simulink model "example_multilateration"  (R2016a)
settings: Solver=VariableStepAuto  StartTime=0.0  StopTime=25  RelTol=1e-3
undefined symbols (not defined in the file): inner_h, k, TDOAparam
libraries: dspsrcs4 x6, vrlib x2
settings Model: Creator=Daniel  LastModifiedBy=mgreiff
settings DataIOCC: LimitDataPoints=on
settings DebuggingCC: AllowSymbolicDim=off
settings ModelReferenceCC: PropagateSignalLabelsOutOfModel=off
settings GRTTargetCC: GeneratePreprocessorConditionals=Use local settings

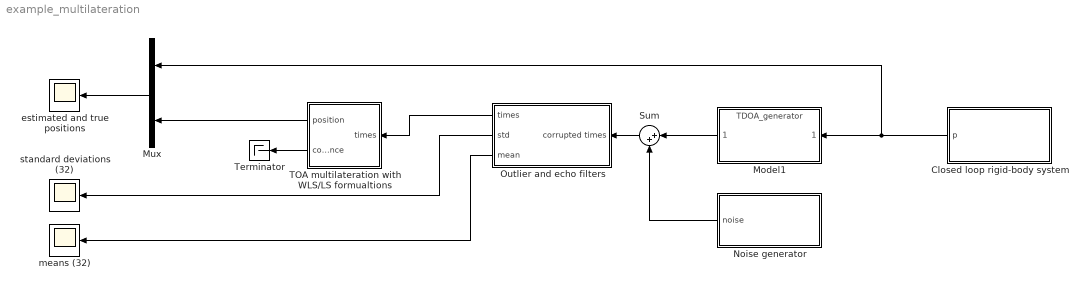
== system example_multilateration ==
  Closed loop rigid-body system : Subsystem
  Model1 : ModelReference  ModelNameDialog=TDOA_generator.slx  SimulationMode=Normal  ModelReferenceVersion=1.3
  Mux : Mux  Inputs=2
  Noise generator : Subsystem
  Outlier and echo filters : Subsystem
  Sum : Sum  Inputs=|++
  TOA multilateration with WLS/LS formualtions : Subsystem
  Terminator : Terminator
  estimated and true positions : Scope
  means (32) : Scope
  standard deviations (32) : Scope
  wires:
  Sum/1 -> Outlier and echo filters/1(corrupted times)
  Outlier and echo filters/2(std) -> standard deviations (32)/1
  Outlier and echo filters/3(mean) -> means (32)/1
  Outlier and echo filters/1(times) -> TOA multilateration with WLS/LS formualtions/1(times)
  TOA multilateration with WLS/LS formualtions/2(confidence) -> Terminator/1
  Closed loop rigid-body system/1(p) -> Mux/1, Model1/1
  Mux/1 -> estimated and true positions/1
  TOA multilateration with WLS/LS formualtions/1(position) -> Mux/2
  Noise generator/1(noise) -> Sum/2
  Model1/1 -> Sum/1

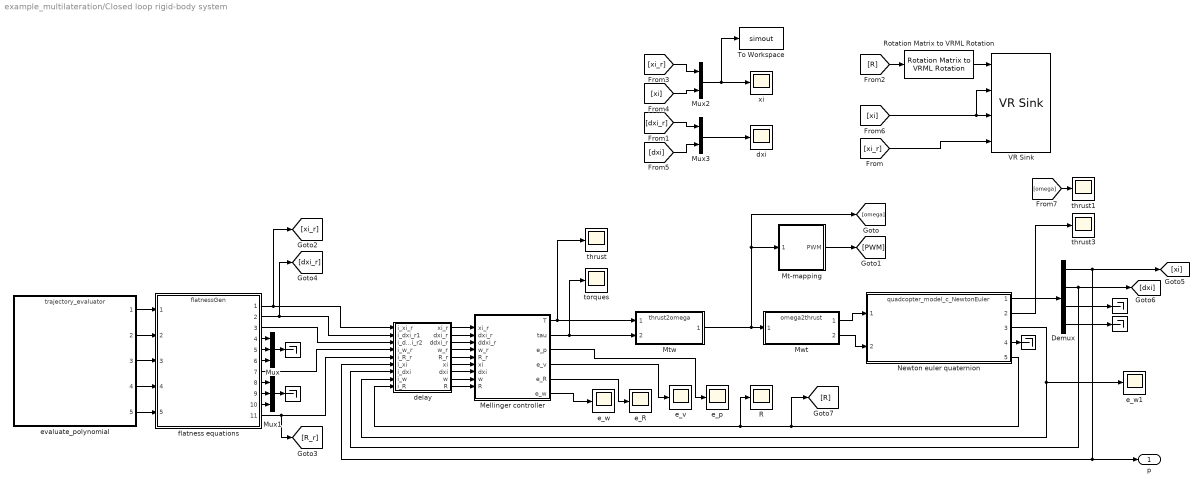
== system example_multilateration/Closed loop rigid-body system ==
  " " : Terminator
  "  " : Terminator
  "     " : Terminator
  "      " : Terminator
  "       " : Terminator
  Demux : Demux  Outputs=[3,3,3,3]
  Mellinger controller : MATLAB Function  TreatAsAtomicUnit=on  SystemSampleTime=inner_h
  Mt-mapping : Subsystem
  Mtw : ModelReference  ModelNameDialog=thrust2omega.mdl  SimulationMode=Normal  ModelReferenceVersion=1.3
  Mux : Mux  Inputs=3
  Mux1 : Mux  Inputs=3
  Mux2 : Mux  Inputs=2
  Mux3 : Mux  Inputs=2
  Mwt : ModelReference  ModelNameDialog=omega2thrust.mdl  SimulationMode=Normal  ModelReferenceVersion=1.3
  Newton euler quaternion : ModelReference  ModelNameDialog=quadcopter_model_c_NewtonEuler.mdl  SimulationMode=Normal  ModelReferenceVersion=1.325
  R : Scope
  Rotation Matrix to VRML Rotation : vrlib/Utilities/Rotation Matrix to VRML Rotation  maxzero=1e-12
  To Workspace : ToWorkspace  VariableName=simout  SaveFormat=Timeseries  SampleTime=-1
  VR Sink : vrlib/VR Sink  InstantiateOnLoad=on  SampleTime=0.05  ViewEnable=on  RemoteChange=off  RemoteView=off  FieldsWritten=copter.rotation.4.1.1.double#copter.translation.3.1.1.double#vp.translation.3.1.1.double#target.translation.3.1.1.double  WorldFileName=copter_world.wrl  WorldDescription=quadcopter_world  AutoView=on  VideoDimensions=[]  AllowVariableSize=off
  delay : Subsystem
  dxi : Scope
  e_R : Scope
  e_p : Scope
  e_v : Scope
  e_w : Scope
  e_w1 : Scope
  evaluate_polynomial : ModelReference  ModelNameDialog=trajectory_evaluator.slx  SimulationMode=Normal  ModelReferenceVersion=1.106
  flatness equations : ModelReference  ModelNameDialog=flatnessGen.slx  SimulationMode=Normal  ModelReferenceVersion=1.117
  thrust : Scope
  thrust1 : Scope
  thrust3 : Scope
  torques : Scope
  xi : Scope
  p : Outport
  wires:
  Demux/4 -> "       "/1
  flatness equations/2 -> delay/2(i_dxi_r1), [dxi_r]
  [xi] -> Mux2/2
  Mux3/1 -> dxi/1
  flatness equations/10 -> Mux1/3
  Mwt/1 -> Newton euler quaternion/1
  Mt-mapping/1(PWM) -> [PWM]
  Mellinger controller/2(tau) -> torques/1, Mtw/2
  delay/7(dxi) -> Mellinger controller/7(dxi)
  evaluate_polynomial/5 -> flatness equations/5
  delay/4(w_r) -> Mellinger controller/4(w_r)
  delay/9(R) -> Mellinger controller/9(R)
  flatness equations/4 -> Mux/1
  delay/3(ddxi_r) -> Mellinger controller/3(ddxi_r)
  delay/1(xi_r) -> Mellinger controller/1(xi_r)
  flatness equations/7 -> delay/4(i_w_r)
  [R] -> Rotation Matrix to VRML Rotation/1
  Mwt/2 -> Newton euler quaternion/2
  evaluate_polynomial/4 -> flatness equations/4
  [dxi] -> Mux3/2
  Mux2/1 -> To Workspace/1, xi/1
  Mux1/1 -> "  "/1
  [xi_r] -> VR Sink/4
  Demux/3 -> "      "/1
  delay/5(R_r) -> Mellinger controller/5(R_r)
  delay/6(xi) -> Mellinger controller/6(xi)
  Newton euler quaternion/5 -> [R], delay/9(i_R), R/1
  Newton euler quaternion/4 -> "     "/1
  evaluate_polynomial/2 -> flatness equations/2
  [dxi_r] -> Mux3/1
  evaluate_polynomial/1 -> flatness equations/1
  Demux/1 -> delay/6(i_xi), p/1, [xi]
  evaluate_polynomial/3 -> flatness equations/3
  Mtw/1 -> Mt-mapping/1(omega), [omega], Mwt/1
  flatness equations/11 -> delay/5(i_R_r), [R_r]
  flatness equations/9 -> Mux1/2
  Newton euler quaternion/1 -> Demux/1
  delay/2(dxi_r) -> Mellinger controller/2(dxi_r)
  Rotation Matrix to VRML Rotation/1 -> VR Sink/1
  Mellinger controller/3(e_p) -> e_p/1
  flatness equations/1 -> delay/1(i_xi_r), [xi_r]
  Newton euler quaternion/3 -> e_w1/1, delay/8(i_w)
  flatness equations/5 -> Mux/2
  delay/8(w) -> Mellinger controller/8(w)
  Mellinger controller/1(T) -> Mtw/1, thrust/1
  Mellinger controller/4(e_v) -> e_v/1
  flatness equations/3 -> delay/3(i_ddxi_r2)
  Newton euler quaternion/2 -> thrust3/1
  Mellinger controller/6(e_w) -> e_w/1
  Demux/2 -> delay/7(i_dxi), [dxi]
  Mellinger controller/5(e_R) -> e_R/1
  flatness equations/6 -> Mux/3
  [xi_r] -> Mux2/1
  [xi] -> VR Sink/2, VR Sink/3
  Mux/1 -> " "/1
  [omega] -> thrust1/1
  flatness equations/8 -> Mux1/1

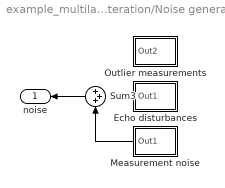
== system example_multilateration/Noise generator ==
  Echo disturbances : Subsystem
  Measurement noise : Subsystem
  Outlier measurements : Subsystem
  Sum3 : Sum  Inputs=+++
  noise : Outport
  wires:
  Sum3/1 -> noise/1
  Measurement noise/1(Out1) -> Sum3/3

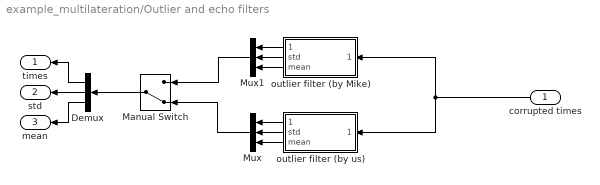
== system example_multilateration/Outlier and echo filters ==
  corrupted times : Inport
  Demux : Demux  Outputs=[6,6,6]
  Manual Switch : ManualSwitch  CurrentSetting=0
  Mux : Mux  Inputs=3
  Mux1 : Mux  Inputs=3
  outlier filter (by Mike) : Subsystem  TreatAsAtomicUnit=on  SystemSampleTime=1/60
  outlier filter (by us) : Subsystem  TreatAsAtomicUnit=on  SystemSampleTime=1/60
  times : Outport
  std : Outport  Port=2
  mean : Outport  Port=3
  wires:
  corrupted times/1 -> outlier filter (by us)/1(tm_tdoa), outlier filter (by Mike)/1(tm_tdoa)
  Manual Switch/1 -> Demux/1
  Mux1/1 -> Manual Switch/1
  outlier filter (by Mike)/1(tf_tdoa) -> Mux1/1
  outlier filter (by Mike)/2(std) -> Mux1/2
  outlier filter (by Mike)/3(mean) -> Mux1/3
  outlier filter (by us)/1(tf_tdoa) -> Mux/1
  outlier filter (by us)/2(std) -> Mux/2
  outlier filter (by us)/3(mean) -> Mux/3
  Mux/1 -> Manual Switch/2
  Demux/3 -> mean/1
  Demux/2 -> std/1
  Demux/1 -> times/1

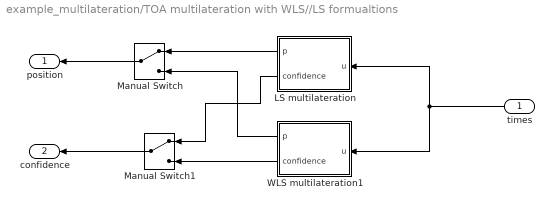
== system example_multilateration/TOA multilateration with WLS//LS formualtions ==
  times : Inport  PortDimensions=6
  LS multilateration : MATLAB Function  TreatAsAtomicUnit=on
  Manual Switch : ManualSwitch
  Manual Switch1 : ManualSwitch
  WLS multilateration1 : MATLAB Function  TreatAsAtomicUnit=on
  position : Outport  PortDimensions=3
  confidence : Outport  Port=2  PortDimensions=3
  wires:
  Manual Switch/1 -> position/1
  times/1 -> WLS multilateration1/1(u), LS multilateration/1(u)
  LS multilateration/1(p) -> Manual Switch/1
  WLS multilateration1/1(p) -> Manual Switch/2
  LS multilateration/2(confidence) -> Manual Switch1/1
  Manual Switch1/1 -> confidence/1
  WLS multilateration1/2(confidence) -> Manual Switch1/2

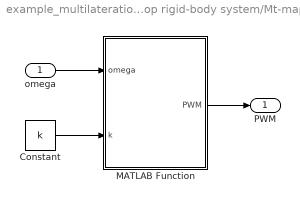
== system example_multilateration/Closed loop rigid-body system/Mt-mapping ==
  omega : Inport
  Constant : Constant  Value=k
  MATLAB Function : MATLAB Function  TreatAsAtomicUnit=on
  PWM : Outport
  wires:
  MATLAB Function/1(PWM) -> PWM/1
  omega/1 -> MATLAB Function/1(omega)
  Constant/1 -> MATLAB Function/2(k)

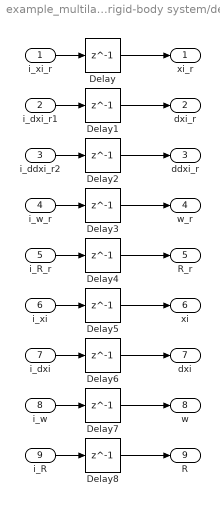
== system example_multilateration/Closed loop rigid-body system/delay ==
  i_xi_r : Inport
  i_dxi_r1 : Inport  Port=2
  i_ddxi_r2 : Inport  Port=3
  i_w_r : Inport  Port=4
  i_R_r : Inport  Port=5
  i_xi : Inport  Port=6
  i_dxi : Inport  Port=7
  i_w : Inport  Port=8
  i_R : Inport  Port=9
  Delay{,1..8} (9 alike) : Delay  DelayLength=1  InitialCondition=0  SampleTime=inner_h
  xi_r : Outport
  dxi_r : Outport  Port=2
  ddxi_r : Outport  Port=3
  w_r : Outport  Port=4
  R_r : Outport  Port=5
  xi : Outport  Port=6
  dxi : Outport  Port=7
  w : Outport  Port=8
  R : Outport  Port=9
  wires:
  Delay/1 -> xi_r/1
  Delay1/1 -> dxi_r/1
  Delay2/1 -> ddxi_r/1
  Delay4/1 -> R_r/1
  Delay3/1 -> w_r/1
  Delay5/1 -> xi/1
  Delay6/1 -> dxi/1
  Delay8/1 -> R/1
  Delay7/1 -> w/1
  i_xi_r/1 -> Delay/1
  i_ddxi_r2/1 -> Delay2/1
  i_dxi_r1/1 -> Delay1/1
  i_w_r/1 -> Delay3/1
  i_R_r/1 -> Delay4/1
  i_xi/1 -> Delay5/1
  i_dxi/1 -> Delay6/1
  i_w/1 -> Delay7/1
  i_R/1 -> Delay8/1

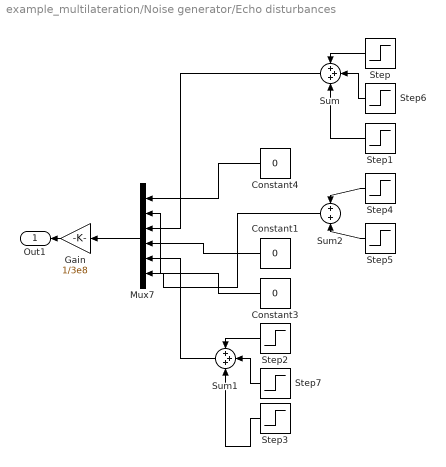
== system example_multilateration/Noise generator/Echo disturbances ==
  Constant1 : Constant  Value=0
  Constant3 : Constant  Value=0
  Constant4 : Constant  Value=0
  Gain : Gain  Gain=1/3e8
  Mux7 : Mux  Inputs=6
  Step : Step  Time=10  After=-0.3  SampleTime=0
  Step1 : Step  Time=14  After=-0.4  SampleTime=0
  Step2 : Step  Time=16  After=0.4  SampleTime=0
  Step3 : Step  Time=22  After=-1  SampleTime=0
  Step4 : Step  Time=3  After=0.3  SampleTime=0
  Step5 : Step  Time=6  After=-0.3  SampleTime=0
  Step6 : Step  Time=12  After=0.7  SampleTime=0
  Step7 : Step  Time=20  After=0.6  SampleTime=0
  Sum : Sum  Inputs=+++
  Sum1 : Sum  Inputs=+++
  Sum2 : Sum  Inputs=+|+
  Out1 : Outport
  wires:
  Step2/1 -> Sum1/1
  Step3/1 -> Sum1/3
  Gain/1 -> Out1/1
  Mux7/1 -> Gain/1
  Step/1 -> Sum/1
  Sum/1 -> Mux7/3
  Constant4/1 -> Mux7/1
  Sum1/1 -> Mux7/5
  Constant3/1 -> Mux7/4
  Constant1/1 -> Mux7/2
  Sum2/1 -> Mux7/6
  Step4/1 -> Sum2/1
  Step5/1 -> Sum2/2
  Step1/1 -> Sum/3
  Step6/1 -> Sum/2
  Step7/1 -> Sum1/2

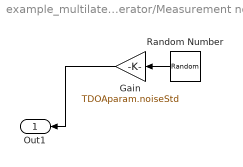
== system example_multilateration/Noise generator/Measurement noise ==
  Gain : Gain  Gain=TDOAparam.noiseStd
  Random Number : RandomNumber  Mean=TDOAparam.noiseMean  Variance=[1,1,1,1,1,1]  SampleTime=1/60
  Out1 : Outport
  wires:
  Gain/1 -> Out1/1
  Random Number/1 -> Gain/1

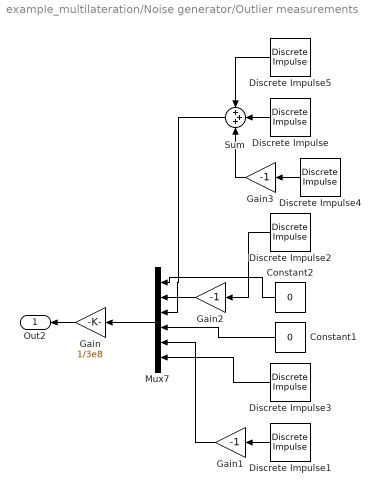
== system example_multilateration/Noise generator/Outlier measurements ==
  Constant1 : Constant  Value=0
  Constant2 : Constant  Value=0
  Discrete Impulse : dspsrcs4/Discrete  Impulse  Delay=700  SampleTime=1/60  FrameSample=1  OutputFrames=off  dataType=double  isSigned=on  wordLen=16  udDataType=sfix(16)  fracBitsMode=Best precision  numFracBits=15  OutDataTypeStr=double  LastOutDataTypeStr=double
  Discrete Impulse1 : dspsrcs4/Discrete  Impulse  Delay=400  SampleTime=1/60  FrameSample=1  OutputFrames=off  dataType=double  isSigned=on  wordLen=16  udDataType=sfix(16)  fracBitsMode=Best precision  numFracBits=15  OutDataTypeStr=double  LastOutDataTypeStr=double
  Discrete Impulse2 : dspsrcs4/Discrete  Impulse  Delay=1000  SampleTime=1/60  FrameSample=1  OutputFrames=off  dataType=double  isSigned=on  wordLen=16  udDataType=sfix(16)  fracBitsMode=Best precision  numFracBits=15  OutDataTypeStr=double  LastOutDataTypeStr=double
  Discrete Impulse3 : dspsrcs4/Discrete  Impulse  Delay=5000  SampleTime=1/60  FrameSample=1  OutputFrames=off  dataType=double  isSigned=on  wordLen=16  udDataType=sfix(16)  fracBitsMode=Best precision  numFracBits=15  OutDataTypeStr=double  LastOutDataTypeStr=double
  Discrete Impulse4 : dspsrcs4/Discrete  Impulse  Delay=800  SampleTime=1/60  FrameSample=1  OutputFrames=off  dataType=double  isSigned=on  wordLen=16  udDataType=sfix(16)  fracBitsMode=Best precision  numFracBits=15  OutDataTypeStr=double  LastOutDataTypeStr=double
  Discrete Impulse5 : dspsrcs4/Discrete  Impulse  Delay=300  SampleTime=1/60  FrameSample=1  OutputFrames=off  dataType=double  isSigned=on  wordLen=16  udDataType=sfix(16)  fracBitsMode=Best precision  numFracBits=15  OutDataTypeStr=double  LastOutDataTypeStr=double
  Gain : Gain  Gain=1/3e8
  Gain1 : Gain  Gain=-1
  Gain2 : Gain  Gain=-1
  Gain3 : Gain  Gain=-1
  Mux7 : Mux  Inputs=6
  Sum : Sum  Inputs=+++
  Out2 : Outport
  wires:
  Gain/1 -> Out2/1
  Discrete Impulse1/1 -> Gain1/1
  Discrete Impulse3/1 -> Mux7/6
  Constant2/1 -> Mux7/1
  Mux7/1 -> Gain/1
  Constant1/1 -> Mux7/4
  Gain1/1 -> Mux7/5
  Gain2/1 -> Mux7/2
  Discrete Impulse2/1 -> Gain2/1
  Discrete Impulse/1 -> Sum/2
  Discrete Impulse4/1 -> Gain3/1
  Discrete Impulse5/1 -> Sum/1
  Sum/1 -> Mux7/3
  Gain3/1 -> Sum/3

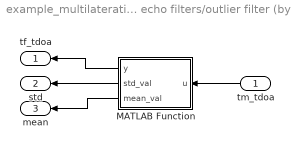
== system example_multilateration/Outlier and echo filters/outlier filter (by Mike) ==
  tm_tdoa : Inport  PortDimensions=6
  MATLAB Function : MATLAB Function  TreatAsAtomicUnit=on
  tf_tdoa : Outport  PortDimensions=6
  std : Outport  Port=2  PortDimensions=6
  mean : Outport  Port=3  PortDimensions=6
  wires:
  MATLAB Function/1(y) -> tf_tdoa/1
  tm_tdoa/1 -> MATLAB Function/1(u)
  MATLAB Function/3(mean_val) -> mean/1
  MATLAB Function/2(std_val) -> std/1

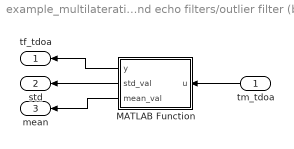
== system example_multilateration/Outlier and echo filters/outlier filter (by us) ==
  tm_tdoa : Inport  PortDimensions=6
  MATLAB Function : MATLAB Function  TreatAsAtomicUnit=on
  tf_tdoa : Outport  PortDimensions=6
  std : Outport  Port=2  PortDimensions=6
  mean : Outport  Port=3  PortDimensions=6
  wires:
  MATLAB Function/1(y) -> tf_tdoa/1
  tm_tdoa/1 -> MATLAB Function/1(u)
  MATLAB Function/3(mean_val) -> mean/1
  MATLAB Function/2(std_val) -> std/1

== matlab function example_multilateration/Outlier and echo filters/outlier filter (by Mike)/MATLAB Function ==
  data: u input; y output; std_val output; mean_val output
function [y, std_val, mean_val] = fcn(u)
persistent TDOA_last_feasible_measurement;
persistent TDOA_series;
if isempty(TDOA_series);
    TDOA_series = zeros(32, 6);
    TDOA_last_feasible_measurement = u;
    disp('here')
end

% Shift TDOA_series such that the most recent measurement is at a low row
% index
TDOA_series(2:end,:) = TDOA_series(1:end-1,:);
TDOA_series(1,:) = u';

series = [];
% Check if the TDOA series contains NaN (cant due ti variable length issues
% in mean() and std())
% if sum(sum(isnan(TDOA_series))) > 0
%     [row, ~] = find(isnan(TDOA_series)); % First column index with NaN
%     series = TDOA_series(1:row(1) - 1, :);
% else
%     series = TDOA_series;
% end

% Compute standard deviation and mean of series;
%if size(series, 1) == 1
std_val = std(TDOA_series);
mean_val = mean(TDOA_series);
   
%end

% 
std_lim = 4;
for ii = 1:length(std_val)
    if std_val(ii)*std_lim >= abs(u(ii) - mean_val(ii))
        TDOA_last_feasible_measurement(ii) = u(ii);
    end
end
y = TDOA_last_feasible_measurement;

== matlab function example_multilateration/Closed loop rigid-body system/Mellinger controller ==
  data: xi_r input; dxi_r input; ddxi_r input; w_r input; R_r input; xi input; T output; tau output; dxi input; w input; R input; e_p output; e_v output; e_R output; e_w output
function [T, tau, e_p, e_v, e_R, e_w] = controller(xi_r, dxi_r, ddxi_r, w_r, R_r, xi, dxi, w, R)
%I = [0.0820; 0.0845; 0.1377];
%A=[0;0;0]
%m = 4.34;

m = 0.027;
g = 9.81;
% Functional tuning for type A
K_p = 0.2 * eye(3);
K_v = 0.025 * eye(3);
K_R = 0.1 * eye(3);
K_w = 0.001 * eye(3);

% Functional tuning for type B
K_p = 0.4 * eye(3);
K_v = 0.1* eye(3);
K_R = 0.4 * eye(3);
K_w = 0.01 * eye(3);

K_p = 0.8 * eye(3);
K_v = 0.12* eye(3);
K_R = 0.5 * eye(3);
K_w = 0.005 * eye(3);

%#codegen
zw = [0; 0; 1];
zb = R(:,3);

e_p = xi_r - xi;
e_v = dxi_r - dxi;
F_des = K_p * e_p + K_v * e_v + m * g * zw + m * ddxi_r;
T = F_des'*zb;

zb_des = F_des./ norm(F_des);
psi = 0;
yc_des = [cos(psi+pi/2); sin(psi+pi/2); 0];
xb_des = cross(yc_des, zb_des)./norm(cross(yc_des, zb_des));
yb_des = cross(zb_des, xb_des);
R_des = [xb_des, yb_des, zb_des];

Ssym = 0.5.* (R_des' * R - R' * R_des);
e_R = -[Ssym(3,2); Ssym(1,3); Ssym(2,1)]; % Vee map
e_w = (w_r - w);

%disp([norm(e_p), norm(e_v), norm(e_R), norm(e_w)])

tau = K_R * e_R + K_w * e_w;

== matlab function example_multilateration/Closed loop rigid-body system/Mt-mapping/MATLAB Function ==
  data: omega input; PWM output; k input
function PWM = Mt(omega, k)
%#codegen
rotor_thrusts = k.*omega.^2;
beta1 = 0.0877;
beta2 = 0.0660;
PWM =  -beta1/(2*beta2) + sqrt((beta1/(2*beta2))^2 + rotor_thrusts/beta2);

== matlab function example_multilateration/Outlier and echo filters/outlier filter (by us)/MATLAB Function ==
  data: u input; y output; std_val output; mean_val output
function [y, std_val, mean_val] = fcn(u)
persistent TDOA_last_feasible_measurement;
persistent TDOA_series;
persistent maxval;
persistent shiftval;
persistent count;
N = 20;
if isempty(TDOA_series);
    TDOA_series = zeros(N, 6);
    TDOA_last_feasible_measurement = u;
    maxval = zeros(1,6);
    shiftval = zeros(1,6);
    count = 0;
end
count = count + 1;

% Shift TDOA_series such that the most recent measurement is at a low row
% index
TDOA_series(2:end,:) = TDOA_series(1:end-1,:);
TDOA_series(1,:) = u';
std_val = zeros(1,6);
mean_val = zeros(1,6);
c = 3e8;

%% Outlier removal in the first five times
limElevation = 0.5/c;
limDiff = 0.2/c;
mean13 = (TDOA_series(1,:) + TDOA_series(3,:))/2;
indicesElevated = abs(mean13 - TDOA_series(2,:)) > limElevation;
indicesClose = abs(TDOA_series(1,:) - TDOA_series(3,:)) < limDiff;
indices = find(indicesElevated + indicesClose > 1);
if ~isempty(indices)
     TDOA_series(2,indices) = mean13(indices);
end

%% Dual series computation
std1 = std(TDOA_series(2:floor(N/2),:));
std2 = std(TDOA_series(ceil(N/2):end,:));
mean1 = mean(TDOA_series(2:floor(N/2),:));
mean2 = mean(TDOA_series(ceil(N/2):end,:));
mean_val = mean1 - mean2;

%% Updates most recent feasible measurements
limStd = 0.1/c;
index1 = std1 < 0.11/c;
index2 = std2 < 0.11/c;
index = index1 + index2;
if sum(index) > 0
    TDOA_last_feasible_measurement(index > 1) = TDOA_series(2,index > 1)';
end

limMean = 0.2/c;
indicesMean = abs(mean_val) > limMean;
std_val = std1;
if count > 100;
    for ii = 1:6
        if indicesMean(ii) > 0 % Above the ii limit
            if abs(maxval(ii)) < abs(mean_val(ii))
                maxval(ii) = mean_val(ii);
            end
        else
            if abs(maxval(ii)) > 0
                shiftval(ii) = shiftval(ii) + maxval(ii);
                maxval(ii) = 0;
            end
        end
    end
end
y = TDOA_last_feasible_measurement - shiftval';

== matlab function example_multilateration/TOA multilateration with WLS//LS formualtions/LS multilateration ==
  data: u input; p output; confidence output
function [p, confidence] = fcn(u)
c = 3e8;
d = u.*c;

sigma = 0.06;

aP = [0,0,2;
      3,0,0;
      6,0,2;
      6,3,0;
      3,3,2;
      0,3,0];

N = 6;
M = N*(N-1)/2;
Sigma = zeros(M,M);
A = zeros(M,3);
b = zeros(M,1);
dP2 = zeros(N,1);

for ii = 1:N
    dP2(ii) = norm(aP(ii,:)).^2;
end

count = 1;
for jj = 1:N;
    for kk = 1:N;
        if jj < kk
            A(count,:) = -2*(aP(jj,:) - aP(kk,:));
            b(count) = (d(jj)^2 - dP2(jj)) - (d(kk)^2 - dP2(kk));
            count = count + 1;
            %Sigma(count,count) TODO fill sigma matrix for confidence
            %intervals
        end
    end
end
p = (A'*A)\(A'*b);
iAA = inv(A'*A);
P = iAA * (A'*Sigma*A) * iAA;
confidence = sqrt(diag(P));

== matlab function example_multilateration/TOA multilateration with WLS//LS formualtions/WLS multilateration1 ==
  data: u input; p output; confidence output
function [p, confidence] = fcn(u)
c = 3e8;
d = u.*c;

stdev = 0.06;

aP = [0,0,2;
      3,0,0;
      6,0,2;
      6,3,0;
      3,3,2;
      0,3,0];

N = 6;
G = zeros(N,4);
c = zeros(N,1);
dP2 = zeros(N,1);

for ii = 1:N
    dP2(ii) = norm(aP(ii,:)).^2;
end

for ii = 1:N;
    G(ii, 1:3) = -2*aP(ii,:);
    G(ii, 4) = 2;
    c(ii) = d(ii)^2 - dP2(ii);
end
W = diag(1./(d.^2));
theta = (G'*W*G)\(G'*W*c);
p = theta(1:3);

Sigma = 4 .* stdev.^2 .* diag(d.^2);
iGWG = inv(G'*W*G);
P = iGWG*(G'*W*Sigma*W*G)*iGWG;
confidence = sqrt(diag(P(1:3,1:3)));
